simulink model "digital_twin_group5"  (R2025a)
settings: Solver=ode1  StartTime=0.0  StopTime=24  FixedStep=1  RelTol=1e-3
libraries: simulink_extras x1
settings Model: Creator=gabeg  LastModifiedBy=gabeg

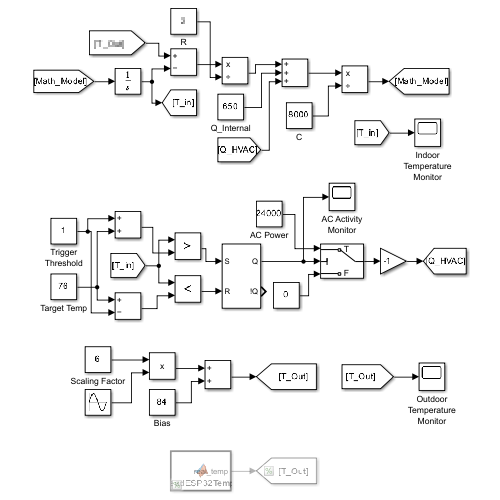
[thumbnail: Simulink's stored preview of the top-level diagram]
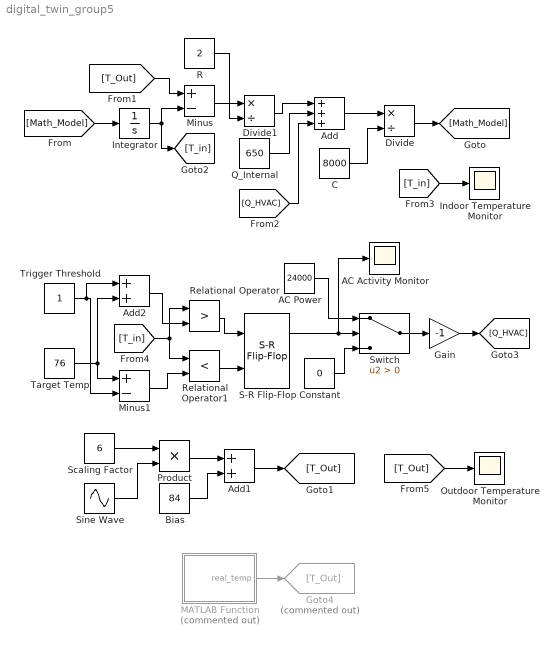
== system digital_twin_group5 ==
  AC Activity Monitor : Scope
      settings: ActiveDisplayYMinimum=-1.4150126871182183  ActiveDisplayYMaximum=2.0861651130914005  DataLoggingVariableName=ScopeData2
  AC Power : Constant  Value=24000
  Add : Sum  Inputs=+++
  Add1 : Sum
  Add2 : Sum
  Bias : Constant  Value=84
  C : Constant  Value=8000
  Constant : Constant  Value=0
  Divide : Product  Inputs=*/
  Divide1 : Product  Inputs=*/
  Gain : Gain  Gain=-1
  Goto4 : Goto  Commented=on  GotoTag=T_Out
  Indoor Temperature Monitor : Scope
      settings: ActiveDisplayYMinimum=76.394801951188938  ActiveDisplayYMaximum=77.297943323390427
  Integrator : Integrator  InitialCondition=75
  MATLAB Function : MATLAB Function  Commented=on  TreatAsAtomicUnit=on
  Minus : Sum  Inputs=+-
  Minus1 : Sum  Inputs=+-
  Outdoor Temperature Monitor : Scope
      settings: ActiveDisplayYMinimum=40.515425165929294  ActiveDisplayYMaximum=109.29389298906798
  Product : Product
  Q_Internal : Constant  Value=650
  R : Constant  Value=2
  Relational Operator : RelationalOperator  Operator=>  OutDataTypeStr=boolean  RndMeth=Simplest  InputSameDT=off
  Relational Operator1 : RelationalOperator  Operator=<  OutDataTypeStr=boolean  RndMeth=Simplest  InputSameDT=off
  S-R Flip-Flop : simulink_extras/Flip Flops/S-R Flip-Flop  initial_condition=0
  Scaling Factor : Constant  Value=6
  Sine Wave : Sin  Frequency=pi/12  Phase=-5*pi/6  SampleTime=0
  Switch : Switch  Criteria=u2 > Threshold  SaturateOnIntegerOverflow=off  InputSameDT=off
  Target Temp : Constant  Value=76
  Trigger Threshold : Constant
  wires:
  Minus/1 -> Divide1/1
  Add/1 -> Divide/1
  Divide/1 -> [Math_Model]
  [Math_Model] -> Integrator/1
  Integrator/1 -> Minus/2, [T_in]
  Sine Wave/1 -> Product/2
  Scaling Factor/1 -> Product/1
  Product/1 -> Add1/1
  Bias/1 -> Add1/2
  Add1/1 -> [T_Out]
  C/1 -> Divide/2
  Q_Internal/1 -> Add/2
  [Q_HVAC] -> Add/3
  [T_in] -> Indoor Temperature Monitor/1
  Trigger Threshold/1 -> Minus1/2, Add2/1
  Target Temp/1 -> Add2/2, Minus1/1
  [T_in] -> Relational Operator1/1, Relational Operator/1
  Add2/1 -> Relational Operator/2
  Minus1/1 -> Relational Operator1/2
  Relational Operator1/1 -> S-R Flip-Flop/2
  Relational Operator/1 -> S-R Flip-Flop/1
  S-R Flip-Flop/1 -> AC Activity Monitor/1, Switch/2
  AC Power/1 -> Switch/1
  Constant/1 -> Switch/3
  Switch/1 -> Gain/1
  Gain/1 -> [Q_HVAC]
  [T_Out] -> Minus/1
  Divide1/1 -> Add/1
  R/1 -> Divide1/2
  [T_Out] -> Outdoor Temperature Monitor/1
  MATLAB Function/1(real_temp) -> Goto4/1

== matlab function digital_twin_group5/MATLAB Function ==
  data: real_temp output
function real_temp = readESP32Temp()
% This block's only job is to call the external helper function.

    % Declare the helper function as extrinsic
    coder.extrinsic('readMySensor');
    
    % Initialize the output for the code generator
    real_temp = 0.0;
    
    % Call the helper function to get the latest temperature
    real_temp = readMySensor();
end
